simulink model "motion_example3"  (Simulink 4.00)
settings: Solver=ode45  StartTime=0.0  StopTime=3  MaxStep=1e-4  RelTol=1e-6  AbsTol=1e-6
values from neighbouring files (symbols this model uses):
  Adff0 = [ 0    1  0   0      0    ((m1+m2)+k1*k2/c)*.5  (m1*k2+m2*k1)/c ... (first row only)    [makeplant.m]
  Bdff0 = [ m1*m2/c/2 ... (first row only)    [makeplant.m]
  Cdff0 = [ 1     0  0   0   (k1+k2)  ((m1+m2)+k1*k2/c)*.5       0 ... (first row only)    [makeplant.m]
  Ddff0 = [  0 ... (first row only)    [makeplant.m]
  Ts = 5e-3    (= 0.005)    [makeplant.m]    (also in profile3.m = acc; recalc.m = 0.001)
undefined symbols (not defined in the file or in its folder): Ac, Acd, Bc, Bcd, Cc, Ccd, Dc, Ddd
libraries: motion x11, simulink3 x5, cstblocks x2
settings Model: LastModifiedBy=plambrec  LimitDataPoints=off  ExtModeTrigMode=oneshot  ExtModeArmWhenConnect=off

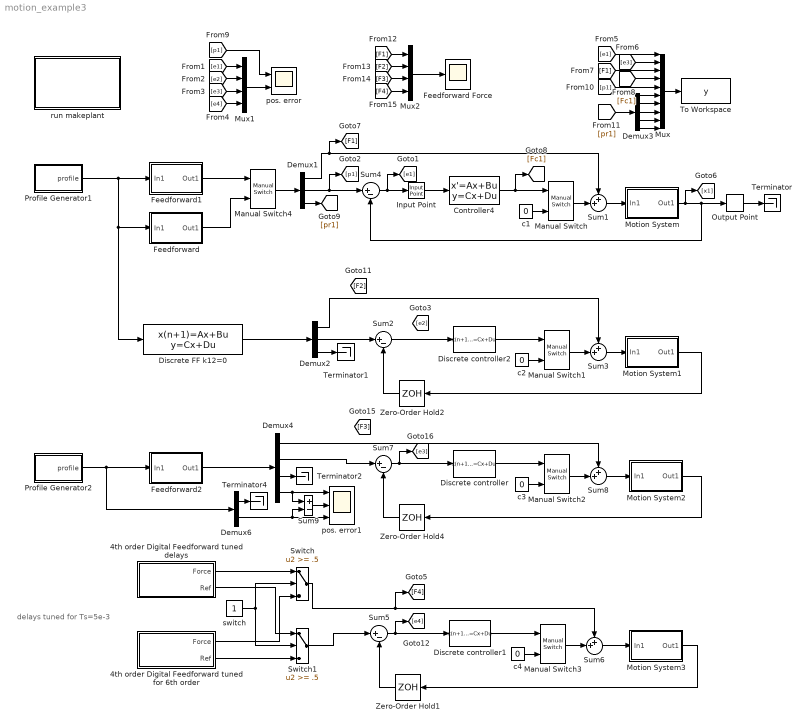
== system motion_example3 ==
  note: delays tuned for Ts=5e-3
  4th order Digital Feedforward tuned delays : Subsystem  mask{t0=.3, x=1, v=1, a=5, j=50, d=1000, Ts=Ts, r=10*eps, s=15, m1=20, m2=10, k1=10, k2=10, c=6.0e5, k12=500}
      mask prompts: t0 "Starting time:  t0 [s]"; x "Displacement:  x [m]"; v "Bound on velocity:  vmax [m/s]"; a "Bound on acceleration:  amax [m/s2]"; j "Bound on jerk: jmax [m/s3]"; d "Bound on derivative of jerk:  dmax [m/s4]"; Ts "Sampling time (0 for continuous):  Ts [s]"; r "Resolution of position [m] (default: 10*eps)"; s "Number of decimals for digitized d (default: 15)"; m1 "Actuator Mass [kg]"; m2 "Load Mass [kg]"; k1 "Actuator to ground Damping [Ns/m]"; k2 "Load to ground Damping [Ns/m]"; c "Spring Stiffness [N/m]"; k12 "Internal Damping [Ns/m]"
      mask init:
      | if length(r)==0 | length(s)==0
      | 	r=10*eps;
      | 	s=15;
      | end
      | [t,dd]=make4(abs(x),v,a,j,d,Ts,r,s);
      | t01=t0-10*eps;
      | if Ts==0
      |    [dj1,tx1,d1,j1,a1,v1,p1,tt1]=profile4(t,dd(1),.001,0);
      | else
      |    [dj1,tx1,d1,j1,a1,v1,p1,tt1]=profile4(t,dd(1),Ts/10,0);
      | end
      settings: RTWFcnNameOpts=Auto  RTWFileNameOpts=Auto
      mask Display:
      | plot([0 dj1(1,:)+t0],[0 dj1(2,:)])
      | text(0.9*(max(dj1(1,:))+t0),0,'F\nx')
  4th order Digital Feedforward tuned for 6th order : Subsystem  mask{t0=.3, x=1, v=1, a=5, j=50, d=1000, Ts=Ts, r=10*eps, s=15, m1=20, m2=10, k1=10, k2=10, c=4.6e5, k12=500}
      mask prompts: t0 "Starting time:  t0 [s]"; x "Displacement:  x [m]"; v "Bound on velocity:  vmax [m/s]"; a "Bound on acceleration:  amax [m/s2]"; j "Bound on jerk: jmax [m/s3]"; d "Bound on derivative of jerk:  dmax [m/s4]"; Ts "Sampling time (0 for continuous):  Ts [s]"; r "Resolution of position [m] (default: 10*eps)"; s "Number of decimals for digitized d (default: 15)"; m1 "Actuator Mass [kg]"; m2 "Load Mass [kg]"; k1 "Actuator to ground Damping [Ns/m]"; k2 "Load to ground Damping [Ns/m]"; c "Spring Stiffness [N/m]"; k12 "Internal Damping [Ns/m]"
      mask init: same as motion_example3/4th order Digital Feedforward tuned delays
      settings: RTWFcnNameOpts=Auto  RTWFileNameOpts=Auto
      mask Display:
      | plot([0 dj1(1,:)+t0],[0 dj1(2,:)])
      | text(0.9*(max(dj1(1,:))+t0),0,'F\nx')
  Controller4 : StateSpace  A=Ac  B=Bc  C=Cc  D=Dc  X0=0  Realization=auto  AbsoluteTolerance=auto
  Demux1 : Demux  Outputs=[1 1 5]  BusSelectionMode=off
  Demux2 : Demux  Outputs=[1 1 4]  BusSelectionMode=off
  Demux3 : Demux  Outputs=5  BusSelectionMode=off
  Demux4 : Demux  Outputs=[1 1 4 1]  BusSelectionMode=off
  Demux6 : Demux  Outputs=2  BusSelectionMode=off
  Discrete FF k12=0 : DiscreteStateSpace  A=Adff0  B=Bdff0  C=Cdff0  D=Ddff0  X0=0  SampleTime=Ts  Realization=auto
  Discrete controller : DiscreteStateSpace  A=Acd  B=Bcd*1.4  C=Ccd  D=Ddd  X0=0  SampleTime=Ts  Realization=auto
  Discrete controller1 : DiscreteStateSpace  A=Acd  B=Bcd*1.4  C=Ccd  D=Ddd  X0=0  SampleTime=Ts  Realization=auto
  Discrete controller2 : DiscreteStateSpace  A=Acd  B=Bcd*1.4  C=Ccd  D=Ddd  X0=0  SampleTime=Ts  Realization=auto
  Feedforward : Subsystem  BlockChoice=4th order continuous
      link override 4th order cont: k1=10  k2=10
      settings: AttributesFormatString=%<BlockChoice>  TemplateBlock=motion/Feedforward Controllers/Feedforward  MemberBlocks=2nd order continuous,2nd order discrete,3d order continuous,3d order discrete,4th order continuous,4th order digital,4th order discrete  RTWFcnNameOpts=Auto  RTWFileNameOpts=Auto
  Feedforward Force : Scope
      settings: TimeRange=3  YMin=-100  YMax=300  SaveToWorkspace=off  SaveName=ScopeData7  LimitDataPoints=on  MaxDataPoints=50000
  Feedforward1 : Subsystem  BlockChoice=4th order continuous
      link override 4th order cont: m1=30  m2=0  k1=20  k2=0  k12=0
      settings: AttributesFormatString=%<BlockChoice>  TemplateBlock=motion/Feedforward Controllers/Feedforward  MemberBlocks=2nd order continuous,2nd order discrete,3d order continuous,3d order discrete,4th order continuous,4th order digital,4th order discrete  RTWFcnNameOpts=Auto  RTWFileNameOpts=Auto
  Feedforward2 : Subsystem  BlockChoice=4th order digital
      link override 4th order digital: r=1e-3
      settings: AttributesFormatString=%<BlockChoice>  TemplateBlock=motion/Feedforward Controllers/Feedforward  MemberBlocks=2nd order continuous,2nd order discrete,3d order continuous,3d order discrete,4th order continuous,4th order digital,4th order discrete  RTWFcnNameOpts=Auto  RTWFileNameOpts=Auto
  Input Point : cstblocks/Input Point
  Manual Switch{,1..4} (5 alike) : simulink3/Nonlinear/Manual Switch  sw=0  action=0
  Motion System : Subsystem  BlockChoice=Parametrized 4th order
      link override Parametrized 4th order: k1=10  k2=10  c=6e5
      settings: AttributesFormatString=%<BlockChoice>  TemplateBlock=motion/Motion Systems1/Motion System  MemberBlocks=2nd order,4th order,6th order,Parametrized 4th order  RTWFcnNameOpts=Auto  RTWFileNameOpts=Auto
  Motion System1 : Subsystem  BlockChoice=Parametrized 4th order
      link override Parametrized 4th order: k1=10  k2=10
      settings: AttributesFormatString=%<BlockChoice>  TemplateBlock=motion/Motion Systems1/Motion System  MemberBlocks=2nd order,4th order,6th order,Parametrized 4th order  RTWFcnNameOpts=Auto  RTWFileNameOpts=Auto
  Motion System2 : Subsystem  BlockChoice=Parametrized 4th order
      link override Parametrized 4th order: k1=10  k2=10
      settings: AttributesFormatString=%<BlockChoice>  TemplateBlock=motion/Motion Systems1/Motion System  MemberBlocks=2nd order,4th order,6th order,Parametrized 4th order  RTWFcnNameOpts=Auto  RTWFileNameOpts=Auto
  Motion System3 : Subsystem  BlockChoice=Parametrized 4th order
      link override Parametrized 4th order: k1=10  k2=10
      settings: AttributesFormatString=%<BlockChoice>  TemplateBlock=motion/Motion Systems1/Motion System  MemberBlocks=2nd order,4th order,6th order,Parametrized 4th order  RTWFcnNameOpts=Auto  RTWFileNameOpts=Auto
  Mux : Mux  Inputs=10
  Mux1 : Mux  Inputs=4
  Mux2 : Mux  Inputs=4
  Output Point : cstblocks/Output Point
  Profile Generator1 : Subsystem  BlockChoice=Derivative of Jerk
      link override Derivative of Jerk: Ts=Ts
      settings: AttributesFormatString=%<BlockChoice>  TemplateBlock=motion/Profile Generators/Profile Generator  MemberBlocks=Acceleration,Derivative of Jerk,Jerk,dJerk with error correction  RTWFcnNameOpts=Auto  RTWFileNameOpts=Auto
  Profile Generator2 : Subsystem  BlockChoice=dJerk with error correction
      link override dJerk with error correction: Ts=Ts  r=1e-3  s=2
      settings: AttributesFormatString=%<BlockChoice>  TemplateBlock=motion/Profile Generators/Profile Generator  MemberBlocks=Acceleration,Derivative of Jerk,Jerk,dJerk with error correction  RTWFcnNameOpts=Auto  RTWFileNameOpts=Auto
  Sum{1,3,6,8} (4 alike) : Sum  Inputs=++|  SaturateOnIntegerOverflow=on
  Sum{2,4..5,7} (4 alike) : Sum  Inputs=|+-  SaturateOnIntegerOverflow=on
  Sum9 : Sum  Inputs=+-  SaturateOnIntegerOverflow=on
  Switch : Switch  Threshold=.5
  Switch1 : Switch  Threshold=.5
  Terminator{,1..2,4} (4 alike) : Terminator
  To Workspace : ToWorkspace  VariableName=y  SampleTime=2e-4  SaveFormat=StructureWithTime
  Zero-Order Hold1 : ZeroOrderHold  Orientation=left  SampleTime=Ts
  Zero-Order Hold2 : ZeroOrderHold  Orientation=left  SampleTime=Ts
  Zero-Order Hold4 : ZeroOrderHold  Orientation=left  SampleTime=Ts
  c{1..4} (4 alike) : Constant  Value=0
  pos. error : Scope  NumInputPorts=2
      settings: TimeRange=3  YMin=0~-8.89489e-008  YMax=1.1~1.0697e-007  SaveToWorkspace=off  SaveName=ScopeData4  LimitDataPoints=on  MaxDataPoints=5000000
  pos. error1 : Scope  NumInputPorts=3
      settings: TimeRange=3  YMin=0~0~-0.006  YMax=1~1.5~0  SaveToWorkspace=off  LimitDataPoints=on  MaxDataPoints=5000000
  run makeplant : Subsystem  ClipboardFcn=edit makeplant
      settings: OpenFcn=makeplant  MoveFcn=edit makeplant  RTWFcnNameOpts=Auto  RTWFileNameOpts=Auto
      mask Display: disp('MAKEPLANT\ndoubleclick to run\nmove to edit')
  switch : Constant  Value=1
  wires:
  Sum1/1 -> Motion System/1(In1)
  Sum4/1 -> Input Point/1, [e1]
  Mux/1 -> To Workspace/1
  Profile Generator1/1(profile) -> Discrete FF k12=0/1, Feedforward/1(In1), Feedforward1/1(In1)
  Output Point/1 -> Terminator/1
  Motion System/1(Out1) -> Output Point/1, Sum4/2, [x1]
  Demux1/2 -> Sum4/1, [p1]
  Demux2/2 -> Sum2/1
  Discrete FF k12=0/1 -> Demux2/1
  Sum3/1 -> Motion System1/1(In1)
  Demux2/1 -> Sum3/1
  Motion System1/1(Out1) -> Zero-Order Hold2/1
  Mux1/1 -> pos. error/2
  Demux1/1 -> [F1], Sum1/1
  Mux2/1 -> Feedforward Force/1
  Demux3/1 -> Mux/6
  Demux3/2 -> Mux/7
  Demux3/3 -> Mux/8
  Demux3/4 -> Mux/9
  Sum2/1 -> Discrete controller2/1
  Demux2/3 -> Terminator1/1
  Zero-Order Hold2/1 -> Sum2/2
  [e1] -> Mux1/1
  [e2] -> Mux1/2
  [e3] -> Mux1/3
  [p1] -> pos. error/1
  [e4] -> Mux1/4
  [e1] -> Mux/1
  [e3] -> Mux/2
  [F1] -> Mux/3
  [Fc1] -> Mux/4
  [p1] -> Mux/5
  Demux1/3 -> [pr1]
  [pr1] -> Demux3/1
  Discrete controller2/1 -> Manual Switch1/1
  c1/1 -> Manual Switch/2
  Controller4/1 -> [Fc1], Manual Switch/1
  Manual Switch/1 -> Sum1/2
  c2/1 -> Manual Switch1/2
  Manual Switch1/1 -> Sum3/2
  [F1] -> Mux2/1
  [F2] -> Mux2/2
  [F3] -> Mux2/3
  [F4] -> Mux2/4
  Sum8/1 -> Motion System2/1(In1)
  Motion System2/1(Out1) -> Zero-Order Hold4/1
  Sum7/1 -> Discrete controller/1, [e3]
  Zero-Order Hold4/1 -> Sum7/2
  Discrete controller/1 -> Manual Switch2/1
  c3/1 -> Manual Switch2/2
  Manual Switch2/1 -> Sum8/2
  Sum6/1 -> Motion System3/1(In1)
  Motion System3/1(Out1) -> Zero-Order Hold1/1
  Sum5/1 -> Discrete controller1/1, [e4]
  Zero-Order Hold1/1 -> Sum5/2
  Discrete controller1/1 -> Manual Switch3/1
  c4/1 -> Manual Switch3/2
  Manual Switch3/1 -> Sum6/2
  Feedforward1/1(Out1) -> Manual Switch4/1
  Manual Switch4/1 -> Demux1/1
  Feedforward/1(Out1) -> Manual Switch4/2
  Input Point/1 -> Controller4/1
  Profile Generator2/1(profile) -> Feedforward2/1(In1), Demux6/1
  Feedforward2/1(Out1) -> Demux4/1
  Demux4/1 -> Sum8/1
  Demux4/2 -> Sum7/1
  switch/1 -> Switch/2, Switch1/2
  4th order Digital Feedforward tuned delays/1(Force) -> Switch/1
  4th order Digital Feedforward tuned delays/2(Ref) -> Switch1/1
  4th order Digital Feedforward tuned for 6th order/1(Force) -> Switch/3
  4th order Digital Feedforward tuned for 6th order/2(Ref) -> Switch1/3
  Switch/1 -> Sum6/1, [F4]
  Switch1/1 -> Sum5/1
  Demux3/5 -> Mux/10
  Demux4/3 -> Terminator2/1
  Demux4/4 -> pos. error1/1, Sum9/1
  Demux6/1 -> Terminator4/1
  Sum9/1 -> pos. error1/2
  Demux6/2 -> Sum9/2, pos. error1/3

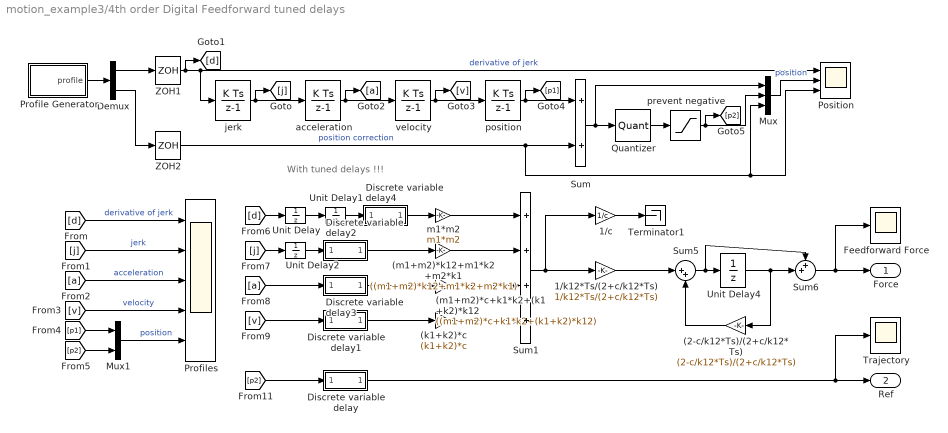
== system motion_example3/4th order Digital Feedforward tuned delays ==
  note: With tuned delays !!!
  (2-c/k12*Ts)/(2+c/k12*Ts) : Gain  Orientation=left  Gain=(2-c/k12*Ts)/(2+c/k12*Ts)  Multiplication=Element-wise(K.*u)  SaturateOnIntegerOverflow=on
  (k1+k2)*c : Gain  Gain=(k1+k2)*c  Multiplication=Element-wise(K.*u)  SaturateOnIntegerOverflow=on
  (m1+m2)*c+k1*k2+(k1+k2)*k12 : Gain  Gain=((m1+m2)*c+k1*k2+(k1+k2)*k12)  Multiplication=Element-wise(K.*u)  SaturateOnIntegerOverflow=on
  (m1+m2)*k12+m1*k2+m2*k1 : Gain  Gain=((m1+m2)*k12+m1*k2+m2*k1)  Multiplication=Element-wise(K.*u)  SaturateOnIntegerOverflow=on
  1/c : Gain  Gain=1/c  Multiplication=Element-wise(K.*u)  SaturateOnIntegerOverflow=on
  1/k12*Ts/(2+c/k12*Ts) : Gain  Gain=1/k12*Ts/(2+c/k12*Ts)  Multiplication=Element-wise(K.*u)  SaturateOnIntegerOverflow=on
  Demux : Demux  Outputs=2  BusSelectionMode=off
  Discrete variable delay : Subsystem  mask{Ts=Ts, alpha=0.5 -0.000278}
      mask prompts: Ts "Sample time"; alpha "Delay factor (between 0 and 1)"
      settings: RTWFcnNameOpts=Auto  RTWFileNameOpts=Auto
      mask Display: disp(sprintf('%3.1f*Ts',alpha))
  Discrete variable delay1 : Subsystem  mask{Ts=Ts, alpha=0.5 -  0.000278}
      mask prompts: Ts "Sample time"; alpha "Delay factor (between 0 and 1)"
      settings: RTWFcnNameOpts=Auto  RTWFileNameOpts=Auto
      mask Display: disp(sprintf('%3.1f*Ts',alpha))
  Discrete variable delay2 : Subsystem  mask{Ts=Ts, alpha=.50}
      mask prompts: Ts "Sample time"; alpha "Delay factor (between 0 and 1)"
      settings: RTWFcnNameOpts=Auto  RTWFileNameOpts=Auto
      mask Display: disp(sprintf('%3.1f*Ts',alpha))
  Discrete variable delay3 : Subsystem  mask{Ts=Ts, alpha=1.00}
      mask prompts: Ts "Sample time"; alpha "Delay factor (between 0 and 1)"
      settings: RTWFcnNameOpts=Auto  RTWFileNameOpts=Auto
      mask Display: disp(sprintf('%3.1f*Ts',alpha))
  Discrete variable delay4 : Subsystem  mask{Ts=Ts, alpha=0 + 0.095}
      mask prompts: Ts "Sample time"; alpha "Delay factor (between 0 and 1)"
      settings: RTWFcnNameOpts=Auto  RTWFileNameOpts=Auto
      mask Display: disp(sprintf('%3.1f*Ts',alpha))
  Feedforward Force : Scope
      settings: TimeRange=3  YMin=-150  YMax=200  SaveToWorkspace=off  SaveName=ScopeData  LimitDataPoints=on  MaxDataPoints=50000
  Mux : Mux  Inputs=3
  Mux1 : Mux  Inputs=2
  Position : Scope  NumInputPorts=3
      settings: TimeRange=3  YMin=-1000~-0.5~-0.0004  YMax=1000~1~0  SaveToWorkspace=off  SaveName=ScopeData2  LimitDataPoints=on  MaxDataPoints=50000
  Profile Generator : Subsystem  BlockChoice=dJerk with error correction
      link override dJerk with error correction: t0=t0  x=x  v=v  a=a  j=j  d=d  Ts=Ts  r=r  s=s
      settings: AttributesFormatString=%<BlockChoice>  TemplateBlock=motion/Profile Generators/Profile Generator  MemberBlocks=Acceleration,Derivative of Jerk,Jerk,dJerk with error correction  RTWFcnNameOpts=Auto  RTWFileNameOpts=Auto
  Profiles : Scope  NumInputPorts=5
      settings: TimeRange=3  YMin=-1000~-50~-5~-7.49453e-017~0  YMax=1000~50~5~1~1  SaveToWorkspace=off  SaveName=ScopeData4  LimitDataPoints=on  MaxDataPoints=50000
  Quantizer : Quantizer  QuantizationInterval=r  LinearizeAsGain=on
  Sum : Sum  Inputs=++  SaturateOnIntegerOverflow=on
  Sum1 : Sum  Inputs=++++  SaturateOnIntegerOverflow=on
  Sum5 : Sum  Inputs=|++  SaturateOnIntegerOverflow=on
  Sum6 : Sum  Inputs=++|  SaturateOnIntegerOverflow=on
  Terminator1 : Terminator
  Trajectory : Scope
      settings: TimeRange=3  YMin=0  YMax=1  SaveToWorkspace=off  SaveName=ScopeData7  LimitDataPoints=on  MaxDataPoints=50000
  Unit Delay{,1..2,4} (4 alike) : UnitDelay  X0=0  SampleTime=Ts
  ZOH1 : ZeroOrderHold  SampleTime=Ts
  ZOH2 : ZeroOrderHold  SampleTime=Ts
  acceleration : DiscreteIntegrator  IntegratorMethod=ForwardEuler  ExternalReset=none  InitialConditionSource=internal  InitialCondition=0  LimitOutput=off  UpperSaturationLimit=inf  LowerSaturationLimit=-inf  ShowSaturationPort=off  ShowStatePort=off  SampleTime=Ts
  jerk : DiscreteIntegrator  IntegratorMethod=ForwardEuler  ExternalReset=none  InitialConditionSource=internal  InitialCondition=0  LimitOutput=off  UpperSaturationLimit=inf  LowerSaturationLimit=-inf  ShowSaturationPort=off  ShowStatePort=off  SampleTime=Ts
  m1*m2 : Gain  Gain=m1*m2  Multiplication=Element-wise(K.*u)  SaturateOnIntegerOverflow=on
  position : DiscreteIntegrator  IntegratorMethod=ForwardEuler  ExternalReset=none  InitialConditionSource=internal  InitialCondition=0  LimitOutput=off  UpperSaturationLimit=inf  LowerSaturationLimit=-inf  ShowSaturationPort=off  ShowStatePort=off  SampleTime=Ts
  "prevent negative " : Saturate  UpperLimit=inf  LowerLimit=0  LinearizeAsGain=on
  velocity : DiscreteIntegrator  IntegratorMethod=ForwardEuler  ExternalReset=none  InitialConditionSource=internal  InitialCondition=0  LimitOutput=off  UpperSaturationLimit=inf  LowerSaturationLimit=-inf  ShowSaturationPort=off  ShowStatePort=off  SampleTime=Ts
  Force : Outport  Port=1
  Ref : Outport  Port=2
  wires:
  Demux/1 -> ZOH1/1
  jerk/1 -> acceleration/1, [j]
  acceleration/1 -> velocity/1, [a]
  velocity/1 -> position/1, [v]
  ZOH1/1 -> jerk/1, Position/1, [d]  "derivative of jerk"
  Demux/2 -> ZOH2/1
  Quantizer/1 -> "prevent negative "/1
  Sum/1 -> Quantizer/1, Mux/1
  Mux/1 -> Position/2  "position"
  position/1 -> Sum/1, [p1]
  ZOH2/1 -> Sum/2, Mux/3, Position/3  "position correction"
  [p1] -> Mux1/1
  [p2] -> Mux1/2
  [d] -> Profiles/1  "derivative of jerk"
  [j] -> Profiles/2  "jerk"
  [a] -> Profiles/3  "acceleration"
  [v] -> Profiles/4  "velocity"
  Mux1/1 -> Profiles/5  "position"
  [d] -> Unit Delay/1
  [j] -> Unit Delay2/1
  [a] -> Discrete variable delay3/1(In1)
  [v] -> Discrete variable delay1/1(In1)
  (m1+m2)*c+k1*k2+(k1+k2)*k12/1 -> Sum1/3
  (k1+k2)*c/1 -> Sum1/4
  Sum1/1 -> 1/c/1, 1/k12*Ts/(2+c/k12*Ts)/1
  [p2] -> Discrete variable delay/1(In1)
  Discrete variable delay/1(Out1) -> Trajectory/1, Ref/1
  "prevent negative "/1 -> Mux/2, [p2]
  Unit Delay/1 -> Unit Delay1/1
  Discrete variable delay4/1(Out1) -> m1*m2/1
  Unit Delay2/1 -> Discrete variable delay2/1(In1)
  Discrete variable delay1/1(Out1) -> (k1+k2)*c/1
  Discrete variable delay2/1(Out1) -> (m1+m2)*k12+m1*k2+m2*k1/1
  1/k12*Ts/(2+c/k12*Ts)/1 -> Sum5/1
  Sum5/1 -> Unit Delay4/1, Sum6/1
  Unit Delay4/1 -> (2-c/k12*Ts)/(2+c/k12*Ts)/1, Sum6/2
  (2-c/k12*Ts)/(2+c/k12*Ts)/1 -> Sum5/2
  Sum6/1 -> Feedforward Force/1, Force/1
  1/c/1 -> Terminator1/1
  (m1+m2)*k12+m1*k2+m2*k1/1 -> Sum1/2
  Profile Generator/1(profile) -> Demux/1
  m1*m2/1 -> Sum1/1
  Discrete variable delay3/1(Out1) -> (m1+m2)*c+k1*k2+(k1+k2)*k12/1
  Unit Delay1/1 -> Discrete variable delay4/1(In1)

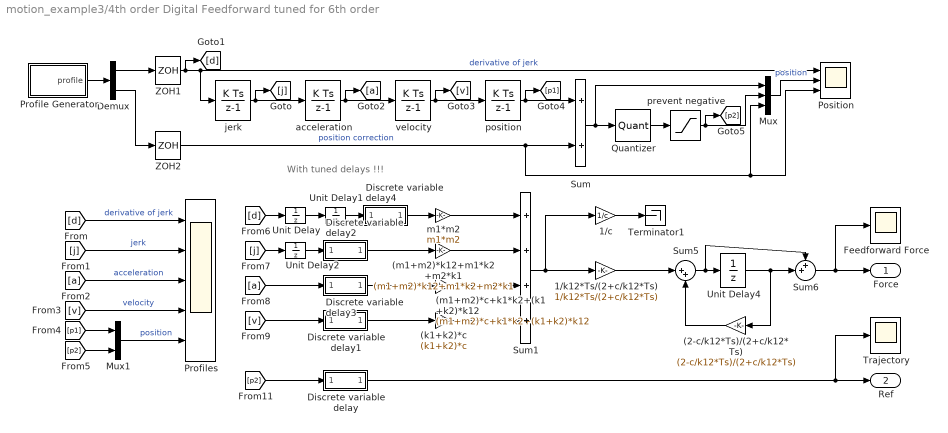
== system motion_example3/4th order Digital Feedforward tuned for 6th order ==
  note: With tuned delays !!!
  (2-c/k12*Ts)/(2+c/k12*Ts) : Gain  Orientation=left  Gain=(2-c/k12*Ts)/(2+c/k12*Ts)  Multiplication=Element-wise(K.*u)  SaturateOnIntegerOverflow=on
  (k1+k2)*c : Gain  Gain=(k1+k2)*c  Multiplication=Element-wise(K.*u)  SaturateOnIntegerOverflow=on
  (m1+m2)*c+k1*k2+(k1+k2)*k12 : Gain  Gain=(m1+m2)*c+k1*k2+(k1+k2)*k12  Multiplication=Element-wise(K.*u)  SaturateOnIntegerOverflow=on
  (m1+m2)*k12+m1*k2+m2*k1 : Gain  Gain=(m1+m2)*k12+m1*k2+m2*k1  Multiplication=Element-wise(K.*u)  SaturateOnIntegerOverflow=on
  1/c : Gain  Gain=1/c  Multiplication=Element-wise(K.*u)  SaturateOnIntegerOverflow=on
  1/k12*Ts/(2+c/k12*Ts) : Gain  Gain=1/k12*Ts/(2+c/k12*Ts)  Multiplication=Element-wise(K.*u)  SaturateOnIntegerOverflow=on
  Demux : Demux  Outputs=2  BusSelectionMode=off
  Discrete variable delay : Subsystem  mask{Ts=Ts, alpha=.4989295}
      mask prompts: Ts "Sample time"; alpha "Delay factor (between 0 and 1)"
      settings: RTWFcnNameOpts=Auto  RTWFileNameOpts=Auto
      mask Display: disp(sprintf('%3.1f*Ts',alpha))
  Discrete variable delay1 : Subsystem  mask{Ts=Ts, alpha=.499726}
      mask prompts: Ts "Sample time"; alpha "Delay factor (between 0 and 1)"
      settings: RTWFcnNameOpts=Auto  RTWFileNameOpts=Auto
      mask Display: disp(sprintf('%3.1f*Ts',alpha))
  Discrete variable delay2 : Subsystem  mask{Ts=Ts, alpha=.4826}
      mask prompts: Ts "Sample time"; alpha "Delay factor (between 0 and 1)"
      settings: RTWFcnNameOpts=Auto  RTWFileNameOpts=Auto
      mask Display: disp(sprintf('%3.1f*Ts',alpha))
  Discrete variable delay3 : Subsystem  mask{Ts=Ts, alpha=1}
      mask prompts: Ts "Sample time"; alpha "Delay factor (between 0 and 1)"
      settings: RTWFcnNameOpts=Auto  RTWFileNameOpts=Auto
      mask Display: disp(sprintf('%3.1f*Ts',alpha))
  Discrete variable delay4 : Subsystem  mask{Ts=Ts, alpha=0.03}
      mask prompts: Ts "Sample time"; alpha "Delay factor (between 0 and 1)"
      settings: RTWFcnNameOpts=Auto  RTWFileNameOpts=Auto
      mask Display: disp(sprintf('%3.1f*Ts',alpha))
  Feedforward Force : Scope
      settings: TimeRange=3  YMin=-150  YMax=200  SaveToWorkspace=off  SaveName=ScopeData  LimitDataPoints=on  MaxDataPoints=50000
  Mux : Mux  Inputs=3
  Mux1 : Mux  Inputs=2
  Position : Scope  NumInputPorts=3
      settings: TimeRange=3  YMin=-1000~-0.5~-0.0004  YMax=1000~1~0  SaveToWorkspace=off  SaveName=ScopeData2  LimitDataPoints=on  MaxDataPoints=50000
  Profile Generator : Subsystem  BlockChoice=dJerk with error correction
      link override dJerk with error correction: t0=t0  x=x  v=v  a=a  j=j  d=d  Ts=Ts  r=r  s=s
      settings: AttributesFormatString=%<BlockChoice>  TemplateBlock=motion/Profile Generators/Profile Generator  MemberBlocks=Acceleration,Derivative of Jerk,Jerk,dJerk with error correction  RTWFcnNameOpts=Auto  RTWFileNameOpts=Auto
  Profiles : Scope  NumInputPorts=5
      settings: TimeRange=3  YMin=-1000~-50~-5~-7.49453e-017~0  YMax=1000~50~5~1~1  SaveToWorkspace=off  SaveName=ScopeData4  LimitDataPoints=on  MaxDataPoints=50000
  Quantizer : Quantizer  QuantizationInterval=r  LinearizeAsGain=on
  Sum : Sum  Inputs=++  SaturateOnIntegerOverflow=on
  Sum1 : Sum  Inputs=++++  SaturateOnIntegerOverflow=on
  Sum5 : Sum  Inputs=|++  SaturateOnIntegerOverflow=on
  Sum6 : Sum  Inputs=++|  SaturateOnIntegerOverflow=on
  Terminator1 : Terminator
  Trajectory : Scope
      settings: TimeRange=3  YMin=0  YMax=1  SaveToWorkspace=off  SaveName=ScopeData7  LimitDataPoints=on  MaxDataPoints=50000
  Unit Delay{,1..2,4} (4 alike) : UnitDelay  X0=0  SampleTime=Ts
  ZOH1 : ZeroOrderHold  SampleTime=Ts
  ZOH2 : ZeroOrderHold  SampleTime=Ts
  acceleration : DiscreteIntegrator  IntegratorMethod=ForwardEuler  ExternalReset=none  InitialConditionSource=internal  InitialCondition=0  LimitOutput=off  UpperSaturationLimit=inf  LowerSaturationLimit=-inf  ShowSaturationPort=off  ShowStatePort=off  SampleTime=Ts
  jerk : DiscreteIntegrator  IntegratorMethod=ForwardEuler  ExternalReset=none  InitialConditionSource=internal  InitialCondition=0  LimitOutput=off  UpperSaturationLimit=inf  LowerSaturationLimit=-inf  ShowSaturationPort=off  ShowStatePort=off  SampleTime=Ts
  m1*m2 : Gain  Gain=m1*m2  Multiplication=Element-wise(K.*u)  SaturateOnIntegerOverflow=on
  position : DiscreteIntegrator  IntegratorMethod=ForwardEuler  ExternalReset=none  InitialConditionSource=internal  InitialCondition=0  LimitOutput=off  UpperSaturationLimit=inf  LowerSaturationLimit=-inf  ShowSaturationPort=off  ShowStatePort=off  SampleTime=Ts
  "prevent negative " : Saturate  UpperLimit=inf  LowerLimit=0  LinearizeAsGain=on
  velocity : DiscreteIntegrator  IntegratorMethod=ForwardEuler  ExternalReset=none  InitialConditionSource=internal  InitialCondition=0  LimitOutput=off  UpperSaturationLimit=inf  LowerSaturationLimit=-inf  ShowSaturationPort=off  ShowStatePort=off  SampleTime=Ts
  Force : Outport  Port=1
  Ref : Outport  Port=2
  wires:
  Unit Delay1/1 -> Discrete variable delay4/1(In1)
  Discrete variable delay3/1(Out1) -> (m1+m2)*c+k1*k2+(k1+k2)*k12/1
  m1*m2/1 -> Sum1/1
  Profile Generator/1(profile) -> Demux/1
  (m1+m2)*k12+m1*k2+m2*k1/1 -> Sum1/2
  1/c/1 -> Terminator1/1
  Sum6/1 -> Force/1, Feedforward Force/1
  (2-c/k12*Ts)/(2+c/k12*Ts)/1 -> Sum5/2
  Unit Delay4/1 -> Sum6/2, (2-c/k12*Ts)/(2+c/k12*Ts)/1
  Sum5/1 -> Sum6/1, Unit Delay4/1
  1/k12*Ts/(2+c/k12*Ts)/1 -> Sum5/1
  Discrete variable delay2/1(Out1) -> (m1+m2)*k12+m1*k2+m2*k1/1
  Discrete variable delay1/1(Out1) -> (k1+k2)*c/1
  Unit Delay2/1 -> Discrete variable delay2/1(In1)
  Discrete variable delay4/1(Out1) -> m1*m2/1
  Unit Delay/1 -> Unit Delay1/1
  "prevent negative "/1 -> [p2], Mux/2
  Discrete variable delay/1(Out1) -> Ref/1, Trajectory/1
  [p2] -> Discrete variable delay/1(In1)
  Sum1/1 -> 1/k12*Ts/(2+c/k12*Ts)/1, 1/c/1
  (k1+k2)*c/1 -> Sum1/4
  (m1+m2)*c+k1*k2+(k1+k2)*k12/1 -> Sum1/3
  [v] -> Discrete variable delay1/1(In1)
  [a] -> Discrete variable delay3/1(In1)
  [j] -> Unit Delay2/1
  [d] -> Unit Delay/1
  Mux1/1 -> Profiles/5  "position"
  [v] -> Profiles/4  "velocity"
  [a] -> Profiles/3  "acceleration"
  [j] -> Profiles/2  "jerk"
  [d] -> Profiles/1  "derivative of jerk"
  [p2] -> Mux1/2
  [p1] -> Mux1/1
  ZOH2/1 -> Position/3, Mux/3, Sum/2  "position correction"
  position/1 -> [p1], Sum/1
  Mux/1 -> Position/2  "position"
  Sum/1 -> Mux/1, Quantizer/1
  Quantizer/1 -> "prevent negative "/1
  Demux/2 -> ZOH2/1
  ZOH1/1 -> [d], Position/1, jerk/1  "derivative of jerk"
  velocity/1 -> [v], position/1
  acceleration/1 -> [a], velocity/1
  jerk/1 -> [j], acceleration/1
  Demux/1 -> ZOH1/1

== system motion_example3/Feedforward ==
  In1 : Inport  Port=1
  4th order continuous : motion/Feedforward Controllers/4th order continuous  m1=20  m2=10  k1=10  k2=10  c=6e5  k12=500
  Out1 : Outport  Port=1
  wires:
  In1/1 -> 4th order continuous/1
  4th order continuous/1 -> Out1/1

== system motion_example3/Feedforward1 ==
  In1 : Inport  Port=1
  4th order continuous : motion/Feedforward Controllers/4th order continuous  m1=20  m2=10  k1=10  k2=10  c=6e5  k12=500
  Out1 : Outport  Port=1
  wires:
  In1/1 -> 4th order continuous/1
  4th order continuous/1 -> Out1/1

== system motion_example3/Feedforward2 ==
  In1 : Inport  Port=1
  4th order digital : motion/Feedforward Controllers/4th order digital  m1=20  m2=10  k1=10  k2=10  c=6e5  k12=500  Ts=Ts  r=1e-3
  Out1 : Outport  Port=1
  wires:
  In1/1 -> 4th order digital/1
  4th order digital/1 -> Out1/1

== system motion_example3/Motion System ==
  In1 : Inport  Port=1
  Parametrized 4th order : motion/Motion Systems1/Parametrized 4th order  m1=20  m2=10  k1=10  k2=10  c=6e5  k12=500
  Out1 : Outport  Port=1
  wires:
  In1/1 -> Parametrized 4th order/1
  Parametrized 4th order/1 -> Out1/1

== system motion_example3/Motion System1 ==
  In1 : Inport  Port=1
  Parametrized 4th order : motion/Motion Systems1/Parametrized 4th order  m1=20  m2=10  k1=10  k2=10  c=6e5  k12=500
  Out1 : Outport  Port=1
  wires:
  In1/1 -> Parametrized 4th order/1
  Parametrized 4th order/1 -> Out1/1

== system motion_example3/Motion System2 ==
  In1 : Inport  Port=1
  Parametrized 4th order : motion/Motion Systems1/Parametrized 4th order  m1=20  m2=10  k1=10  k2=10  c=6e5  k12=500
  Out1 : Outport  Port=1
  wires:
  In1/1 -> Parametrized 4th order/1
  Parametrized 4th order/1 -> Out1/1

== system motion_example3/Motion System3 ==
  In1 : Inport  Port=1
  Parametrized 4th order : motion/Motion Systems1/Parametrized 4th order  m1=20  m2=10  k1=10  k2=10  c=6e5  k12=500
  Out1 : Outport  Port=1
  wires:
  In1/1 -> Parametrized 4th order/1
  Parametrized 4th order/1 -> Out1/1

== system motion_example3/Profile Generator1 ==
  Derivative of Jerk : motion/Profile Generators/Derivative of Jerk  AncestorBlock=library/Derivative of jerk profile generator  t0=.3  x=1  v=1  a=5  j=50  d=1000  Ts=Ts
  profile : Outport  Port=1
  wires:
  Derivative of Jerk/1 -> profile/1

== system motion_example3/Profile Generator2 ==
  dJerk with error correction : motion/Profile Generators/dJerk with error correction  t0=.3  x=1  v=1  a=5  j=50  d=1000  Ts=Ts  r=1e-3  s=2
  profile : Outport  Port=1
  wires:
  dJerk with error correction/1 -> profile/1

== system motion_example3/run makeplant ==
  note: Run makeplant

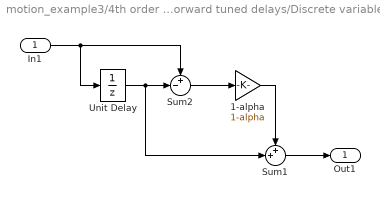
== system motion_example3/4th order Digital Feedforward tuned delays/Discrete variable delay ==
  In1 : Inport  Port=1
  1-alpha : Gain  Gain=1-alpha  Multiplication=Element-wise(K.*u)  SaturateOnIntegerOverflow=on
  Sum1 : Sum  Inputs=++|  SaturateOnIntegerOverflow=on
  Sum2 : Sum  Inputs=+-|  SaturateOnIntegerOverflow=on
  Unit Delay : UnitDelay  X0=0  SampleTime=Ts
  Out1 : Outport  Port=1
  wires:
  In1/1 -> Sum2/1, Unit Delay/1
  Unit Delay/1 -> Sum1/2, Sum2/2
  Sum1/1 -> Out1/1
  1-alpha/1 -> Sum1/1
  Sum2/1 -> 1-alpha/1

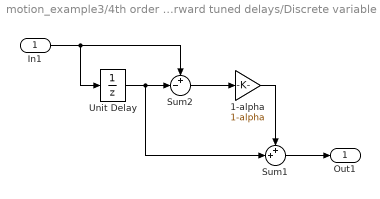
== system motion_example3/4th order Digital Feedforward tuned delays/Discrete variable delay1 ==
  In1 : Inport  Port=1
  1-alpha : Gain  Gain=1-alpha  Multiplication=Element-wise(K.*u)  SaturateOnIntegerOverflow=on
  Sum1 : Sum  Inputs=++|  SaturateOnIntegerOverflow=on
  Sum2 : Sum  Inputs=+-|  SaturateOnIntegerOverflow=on
  Unit Delay : UnitDelay  X0=0  SampleTime=Ts
  Out1 : Outport  Port=1
  wires:
  Sum2/1 -> 1-alpha/1
  1-alpha/1 -> Sum1/1
  Sum1/1 -> Out1/1
  Unit Delay/1 -> Sum2/2, Sum1/2
  In1/1 -> Unit Delay/1, Sum2/1

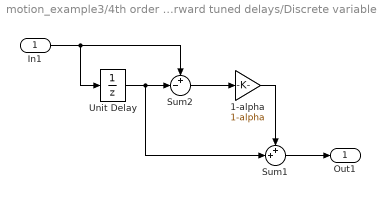
== system motion_example3/4th order Digital Feedforward tuned delays/Discrete variable delay2 ==
  In1 : Inport  Port=1
  1-alpha : Gain  Gain=1-alpha  Multiplication=Element-wise(K.*u)  SaturateOnIntegerOverflow=on
  Sum1 : Sum  Inputs=++|  SaturateOnIntegerOverflow=on
  Sum2 : Sum  Inputs=+-|  SaturateOnIntegerOverflow=on
  Unit Delay : UnitDelay  X0=0  SampleTime=Ts
  Out1 : Outport  Port=1
  wires:
  In1/1 -> Sum2/1, Unit Delay/1
  Unit Delay/1 -> Sum1/2, Sum2/2
  Sum1/1 -> Out1/1
  1-alpha/1 -> Sum1/1
  Sum2/1 -> 1-alpha/1

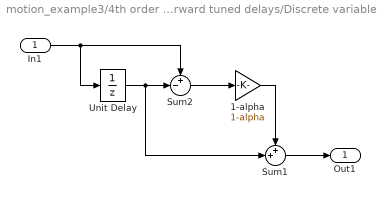
== system motion_example3/4th order Digital Feedforward tuned delays/Discrete variable delay3 ==
  In1 : Inport  Port=1
  1-alpha : Gain  Gain=1-alpha  Multiplication=Element-wise(K.*u)  SaturateOnIntegerOverflow=on
  Sum1 : Sum  Inputs=++|  SaturateOnIntegerOverflow=on
  Sum2 : Sum  Inputs=+-|  SaturateOnIntegerOverflow=on
  Unit Delay : UnitDelay  X0=0  SampleTime=Ts
  Out1 : Outport  Port=1
  wires:
  In1/1 -> Sum2/1, Unit Delay/1
  Unit Delay/1 -> Sum1/2, Sum2/2
  Sum1/1 -> Out1/1
  1-alpha/1 -> Sum1/1
  Sum2/1 -> 1-alpha/1

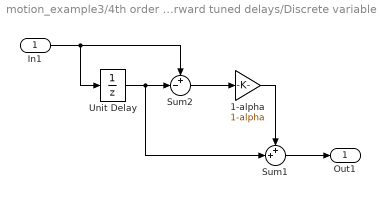
== system motion_example3/4th order Digital Feedforward tuned delays/Discrete variable delay4 ==
  In1 : Inport  Port=1
  1-alpha : Gain  Gain=1-alpha  Multiplication=Element-wise(K.*u)  SaturateOnIntegerOverflow=on
  Sum1 : Sum  Inputs=++|  SaturateOnIntegerOverflow=on
  Sum2 : Sum  Inputs=+-|  SaturateOnIntegerOverflow=on
  Unit Delay : UnitDelay  X0=0  SampleTime=Ts
  Out1 : Outport  Port=1
  wires:
  Sum2/1 -> 1-alpha/1
  1-alpha/1 -> Sum1/1
  Sum1/1 -> Out1/1
  Unit Delay/1 -> Sum2/2, Sum1/2
  In1/1 -> Unit Delay/1, Sum2/1

== system motion_example3/4th order Digital Feedforward tuned delays/Profile Generator ==
  dJerk with error correction : motion/Profile Generators/dJerk with error correction  t0=t0  x=x  v=v  a=a  j=j  d=d  Ts=Ts  r=r  s=s
  profile : Outport  Port=1
  wires:
  dJerk with error correction/1 -> profile/1

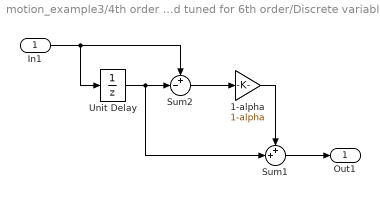
== system motion_example3/4th order Digital Feedforward tuned for 6th order/Discrete variable delay ==
  In1 : Inport  Port=1
  1-alpha : Gain  Gain=1-alpha  Multiplication=Element-wise(K.*u)  SaturateOnIntegerOverflow=on
  Sum1 : Sum  Inputs=++|  SaturateOnIntegerOverflow=on
  Sum2 : Sum  Inputs=+-|  SaturateOnIntegerOverflow=on
  Unit Delay : UnitDelay  X0=0  SampleTime=Ts
  Out1 : Outport  Port=1
  wires:
  Sum2/1 -> 1-alpha/1
  1-alpha/1 -> Sum1/1
  Sum1/1 -> Out1/1
  Unit Delay/1 -> Sum2/2, Sum1/2
  In1/1 -> Unit Delay/1, Sum2/1

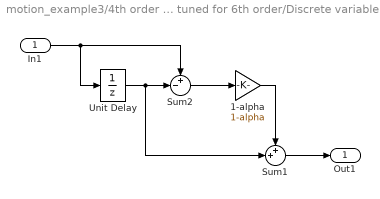
== system motion_example3/4th order Digital Feedforward tuned for 6th order/Discrete variable delay1 ==
  In1 : Inport  Port=1
  1-alpha : Gain  Gain=1-alpha  Multiplication=Element-wise(K.*u)  SaturateOnIntegerOverflow=on
  Sum1 : Sum  Inputs=++|  SaturateOnIntegerOverflow=on
  Sum2 : Sum  Inputs=+-|  SaturateOnIntegerOverflow=on
  Unit Delay : UnitDelay  X0=0  SampleTime=Ts
  Out1 : Outport  Port=1
  wires:
  In1/1 -> Sum2/1, Unit Delay/1
  Unit Delay/1 -> Sum1/2, Sum2/2
  Sum1/1 -> Out1/1
  1-alpha/1 -> Sum1/1
  Sum2/1 -> 1-alpha/1

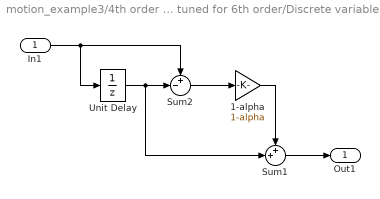
== system motion_example3/4th order Digital Feedforward tuned for 6th order/Discrete variable delay2 ==
  In1 : Inport  Port=1
  1-alpha : Gain  Gain=1-alpha  Multiplication=Element-wise(K.*u)  SaturateOnIntegerOverflow=on
  Sum1 : Sum  Inputs=++|  SaturateOnIntegerOverflow=on
  Sum2 : Sum  Inputs=+-|  SaturateOnIntegerOverflow=on
  Unit Delay : UnitDelay  X0=0  SampleTime=Ts
  Out1 : Outport  Port=1
  wires:
  Sum2/1 -> 1-alpha/1
  1-alpha/1 -> Sum1/1
  Sum1/1 -> Out1/1
  Unit Delay/1 -> Sum2/2, Sum1/2
  In1/1 -> Unit Delay/1, Sum2/1

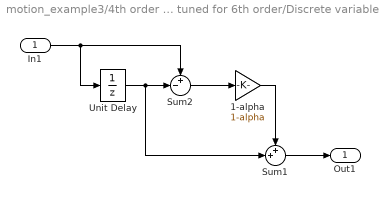
== system motion_example3/4th order Digital Feedforward tuned for 6th order/Discrete variable delay3 ==
  In1 : Inport  Port=1
  1-alpha : Gain  Gain=1-alpha  Multiplication=Element-wise(K.*u)  SaturateOnIntegerOverflow=on
  Sum1 : Sum  Inputs=++|  SaturateOnIntegerOverflow=on
  Sum2 : Sum  Inputs=+-|  SaturateOnIntegerOverflow=on
  Unit Delay : UnitDelay  X0=0  SampleTime=Ts
  Out1 : Outport  Port=1
  wires:
  Sum2/1 -> 1-alpha/1
  1-alpha/1 -> Sum1/1
  Sum1/1 -> Out1/1
  Unit Delay/1 -> Sum2/2, Sum1/2
  In1/1 -> Unit Delay/1, Sum2/1

== system motion_example3/4th order Digital Feedforward tuned for 6th order/Discrete variable delay4 ==
  In1 : Inport  Port=1
  1-alpha : Gain  Gain=1-alpha  Multiplication=Element-wise(K.*u)  SaturateOnIntegerOverflow=on
  Sum1 : Sum  Inputs=++|  SaturateOnIntegerOverflow=on
  Sum2 : Sum  Inputs=+-|  SaturateOnIntegerOverflow=on
  Unit Delay : UnitDelay  X0=0  SampleTime=Ts
  Out1 : Outport  Port=1
  wires:
  In1/1 -> Sum2/1, Unit Delay/1
  Unit Delay/1 -> Sum1/2, Sum2/2
  Sum1/1 -> Out1/1
  1-alpha/1 -> Sum1/1
  Sum2/1 -> 1-alpha/1

== system motion_example3/4th order Digital Feedforward tuned for 6th order/Profile Generator ==
  dJerk with error correction : motion/Profile Generators/dJerk with error correction  t0=t0  x=x  v=v  a=a  j=j  d=d  Ts=Ts  r=r  s=s
  profile : Outport  Port=1
  wires:
  dJerk with error correction/1 -> profile/1
